simulink model "sen_atk_2_sig"  (R2021a)
settings: Solver=VariableStepAuto  StartTime=0.0  StopTime=30  RelTol=1e-3
settings Model: Creator=Suman  LastModifiedBy=Suman

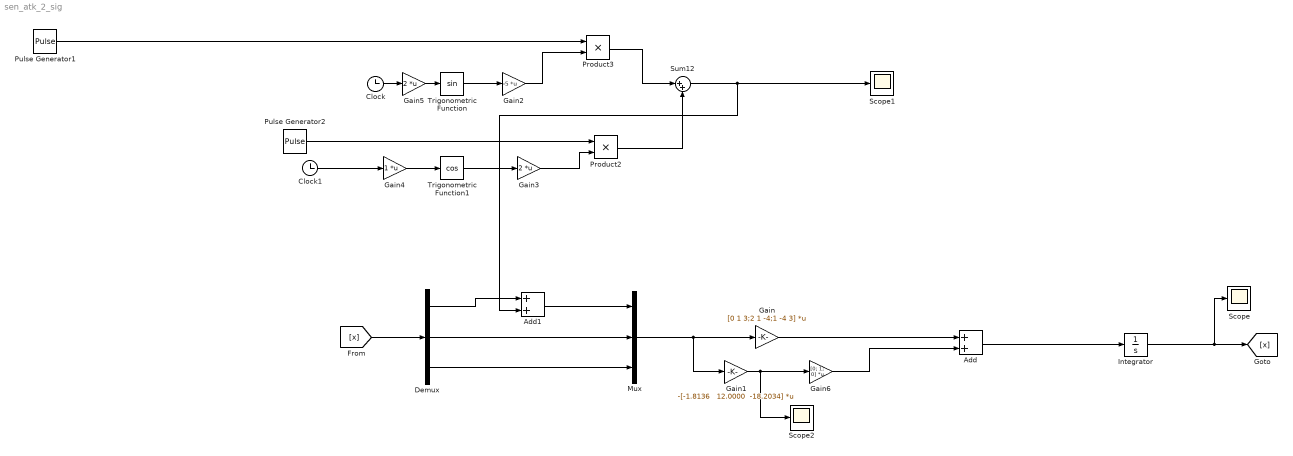
== system sen_atk_2_sig ==
  Add : Sum
  Add1 : Sum
  Clock : Clock
  Clock1 : Clock
  Demux : Demux  Outputs=3
  Gain : Gain  Gain=[0 1 3;2 1 -4;1 -4 3]  Multiplication=Matrix(K*u) (u vector)
  Gain1 : Gain  Gain="-[-1.8136   12.0000  -18.2034]"  Multiplication=Matrix(K*u) (u vector)
  Gain2 : Gain  Gain=-5  Multiplication=Matrix(K*u) (u vector)
  Gain3 : Gain  Gain=2  Multiplication=Matrix(K*u) (u vector)
  Gain4 : Gain  Multiplication=Matrix(K*u) (u vector)
  Gain5 : Gain  Gain=2  Multiplication=Matrix(K*u) (u vector)
  Gain6 : Gain  Gain=[0; 1; 0]  Multiplication=Matrix(K*u)
  Integrator : Integrator  InitialCondition=[2;3;1]
  Mux : Mux  Inputs=3
  Product2 : Product
  Product3 : Product
  Pulse Generator1 : DiscretePulseGenerator  PulseType=Time based  Period=30  PulseWidth=10  PhaseDelay=10
  Pulse Generator2 : DiscretePulseGenerator  PulseType=Time based  Period=30  PulseWidth=10  PhaseDelay=20
  Scope : Scope
  Scope1 : Scope
  Scope2 : Scope
  Sum12 : Sum  Inputs=|++
  Trigonometric Function : Trigonometry
  Trigonometric Function1 : Trigonometry  Operator=cos
  wires:
  Gain5/1 -> Trigonometric Function/1
  Clock1/1 -> Gain4/1
  Add/1 -> Integrator/1
  Product3/1 -> Sum12/1
  Gain4/1 -> Trigonometric Function1/1
  Sum12/1 -> Add1/2, Scope1/1
  Gain/1 -> Add/1
  Product2/1 -> Sum12/2
  Trigonometric Function/1 -> Gain2/1
  Gain3/1 -> Product2/2
  Gain2/1 -> Product3/2
  Trigonometric Function1/1 -> Gain3/1
  Clock/1 -> Gain5/1
  Integrator/1 -> Scope/1, [x]
  Pulse Generator1/1 -> Product3/1
  [x] -> Demux/1
  Mux/1 -> Gain1/1, Gain/1
  Demux/2 -> Mux/2
  Demux/3 -> Mux/3
  Demux/1 -> Add1/1
  Add1/1 -> Mux/1
  Gain1/1 -> Scope2/1, Gain6/1
  Gain6/1 -> Add/2
  Pulse Generator2/1 -> Product2/1
